simulink model "RBD"  (R2022a)
settings: Solver=VariableStepAuto  StartTime=0.0  StopTime=10.0  RelTol=1e-3
undefined symbols (not defined in the file or in its folder): dragConstants, g, J, J_inv, m, projectionMatrix
libraries: matrix_library x1, aerolibutil x1, sharedtransform x1
settings Model: Creator=Drew Lab Computer 1  LastModifiedBy=Drew Lab Computer 1

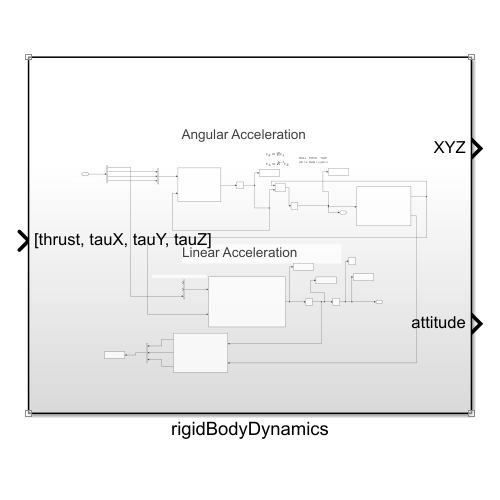
[thumbnail: Simulink's stored preview of the top-level diagram]
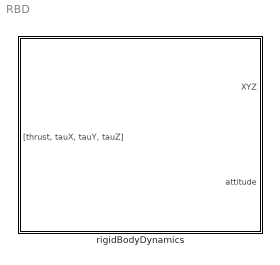
== system RBD ==
  rigidBodyDynamics : Subsystem

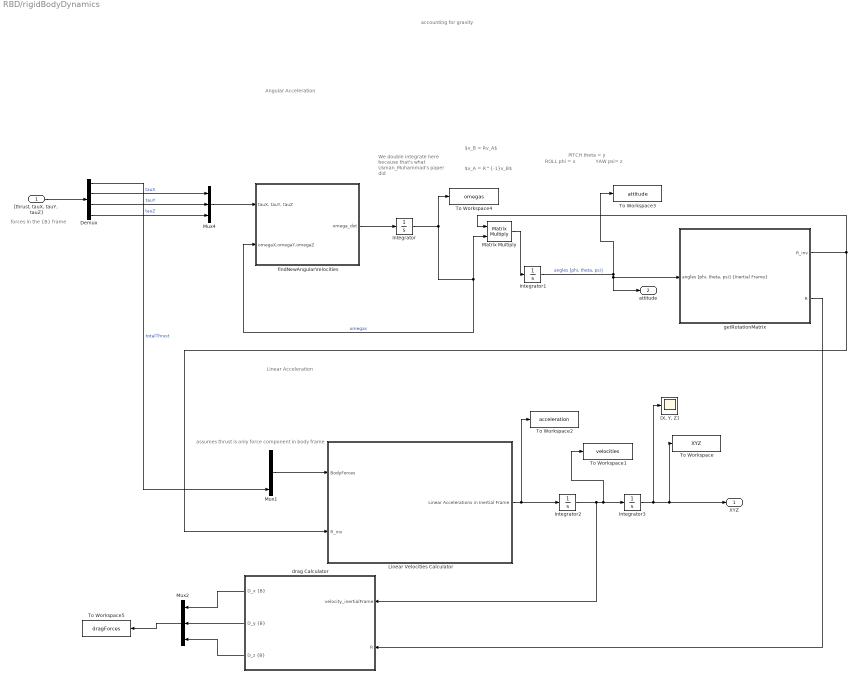
== system RBD/rigidBodyDynamics ==
  note: $v_A = R^{-1}v_B$
  note: assumes thrust is only force component in body frame
  note: We double integrate here because that's what Usman_Muhammad's paper did
  note: Angular Acceleration
  note: Linear Acceleration
  note: accounting for gravity
  note: forces in the {B} frame
  note: ROLL
      | phi = x
  note: PITCH
      | theta = y
  note: YAW
      | psi= z
  note: $v_B = Rv_A$
  "[thrust, tauX, tauY, tauZ]" : Inport
  Demux : Demux
  Integrator{,1..3} (4 alike) : Integrator
  Linear Velocities Calculator : Subsystem
  Matrix Multiply : Product  Multiplication=Matrix(*)
  Mux1 : Mux  Inputs=3
  Mux2 : Mux  Inputs=3
  Mux4 : Mux  Inputs=3
  To Workspace : ToWorkspace  VariableName=XYZ  SaveFormat=Timeseries  SampleTime=-1
  To Workspace1 : ToWorkspace  VariableName=velocities  SaveFormat=Timeseries  SampleTime=-1
  To Workspace2 : ToWorkspace  VariableName=acceleration  SaveFormat=Timeseries  SampleTime=-1
  To Workspace3 : ToWorkspace  VariableName=attitude  SaveFormat=Timeseries  SampleTime=-1
  To Workspace4 : ToWorkspace  VariableName=omegas  SaveFormat=Timeseries  SampleTime=-1
  To Workspace5 : ToWorkspace  VariableName=dragForces  SaveFormat=Timeseries  SampleTime=-1
  "[X, Y, Z]" : Scope
  drag Calculator : Subsystem
  findNewAngularVelocities : Subsystem
  getRotationMatrix : Subsystem
  XYZ : Outport
  attitude : Outport  Port=2
  wires:
  Demux/2 -> Mux4/1  "tauX"
  Demux/4 -> Mux4/3  "tauZ"
  Demux/3 -> Mux4/2  "tauY"
  "[thrust, tauX, tauY, tauZ]"/1 -> Demux/1
  Integrator1/1 -> attitude/1, getRotationMatrix/1("angles [phi, theta, psi] {Inertial Frame}"), To Workspace3/1  "angles [phi, theta, psi]"
  findNewAngularVelocities/1(omega_dot) -> Integrator/1
  Integrator/1 -> Matrix Multiply/2, findNewAngularVelocities/2(omegaX,omegaY,omegaZ), To Workspace4/1  "omegas"
  Mux4/1 -> findNewAngularVelocities/1("tauX, tauY, tauZ")
  Mux1/1 -> Linear Velocities Calculator/1(BodyForces)
  getRotationMatrix/1(R_inv) -> Linear Velocities Calculator/2(R_inv), Matrix Multiply/1
  Demux/1 -> Mux1/3  "totalThrust"
  Matrix Multiply/1 -> Integrator1/1
  Linear Velocities Calculator/1(Linear Accelerations in Inertial Frame) -> Integrator2/1, To Workspace2/1
  Integrator2/1 -> drag Calculator/1(velocity_inertialFrame), To Workspace1/1, Integrator3/1
  Integrator3/1 -> "[X, Y, Z]"/1, To Workspace/1, XYZ/1
  getRotationMatrix/2(R) -> drag Calculator/2(R)
  drag Calculator/2("D_y {B}") -> Mux2/2
  drag Calculator/1("D_x {B}") -> Mux2/1
  drag Calculator/3("D_z {B}") -> Mux2/3
  Mux2/1 -> To Workspace5/1

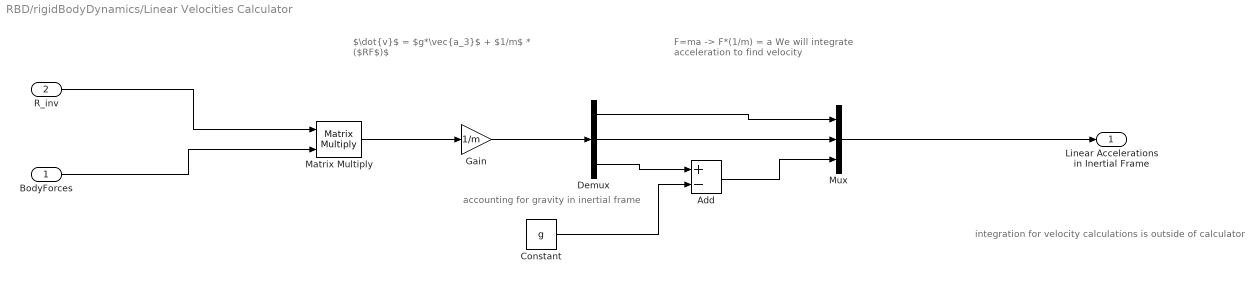
== system RBD/rigidBodyDynamics/Linear Velocities Calculator ==
  note: integration for velocity calculations is outside of calculator
  note: F=ma -> F*(1/m) = a
      | We will integrate acceleration to find velocity
  note: accounting for gravity in inertial frame
  note: $\dot{v}$ = $g*\vec{a_3}$ + $1/m$ * ($RF$)$
  BodyForces : Inport
  R_inv : Inport  Port=2
  Add : Sum  Inputs=+-
  Constant : Constant  Value=g
  Demux : Demux  Outputs=3
  Gain : Gain  Gain=1/m
  Matrix Multiply : Product  Multiplication=Matrix(*)
  Mux : Mux  Inputs=3
  Linear Accelerations in Inertial Frame : Outport
  wires:
  BodyForces/1 -> Matrix Multiply/2
  R_inv/1 -> Matrix Multiply/1
  Matrix Multiply/1 -> Gain/1
  Gain/1 -> Demux/1
  Demux/3 -> Add/1
  Add/1 -> Mux/3
  Demux/2 -> Mux/2
  Demux/1 -> Mux/1
  Mux/1 -> Linear Accelerations in Inertial Frame/1
  Constant/1 -> Add/2

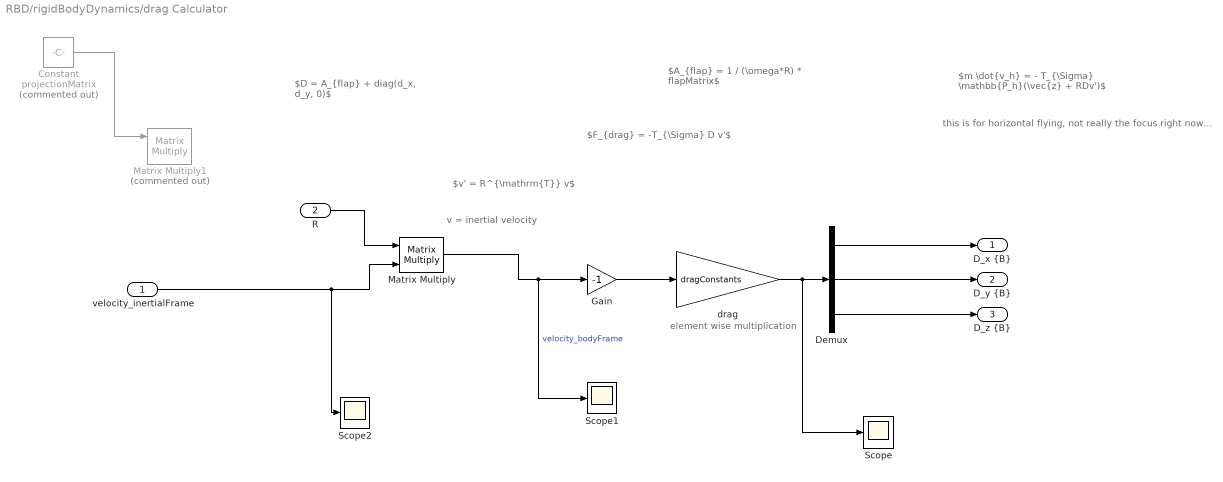
== system RBD/rigidBodyDynamics/drag Calculator ==
  note: element wise multiplication
  note: $A_{flap} = 1 / (\omega*R) * flapMatrix$
  note: $D = A_{flap} + diag(d_x, d_y, 0)$
  note: this is for horizontal flying, not really the focus right now...
  note: $F_{drag} = -T_{\Sigma} D v'$
  note: v = inertial velocity
  note: $v' = R^{\mathrm{T}} v$
  note: $m \dot{v_h} = - T_{\Sigma} \mathbb{P_h}(\vec{z} + RDv')$
  velocity_inertialFrame : Inport
  R : Inport  Port=2
  Constant : Constant  Commented=on  Value=projectionMatrix
  Demux : Demux  Outputs=3
  Gain : Gain  Gain=-1
  Matrix Multiply : Product  Multiplication=Matrix(*)
  Matrix Multiply1 : Product  Commented=on  Multiplication=Matrix(*)
  Scope : Scope
  Scope1 : Scope
  Scope2 : Scope
  drag : Gain  Gain=dragConstants
  "D_x {B}" : Outport
  "D_y {B}" : Outport  Port=2
  "D_z {B}" : Outport  Port=3
  wires:
  Matrix Multiply/1 -> Scope1/1, Gain/1  "velocity_bodyFrame"
  R/1 -> Matrix Multiply/1
  Demux/1 -> "D_x {B}"/1
  Demux/3 -> "D_z {B}"/1
  Gain/1 -> drag/1
  Constant/1 -> Matrix Multiply1/1
  drag/1 -> Scope/1, Demux/1
  Demux/2 -> "D_y {B}"/1
  velocity_inertialFrame/1 -> Scope2/1, Matrix Multiply/2

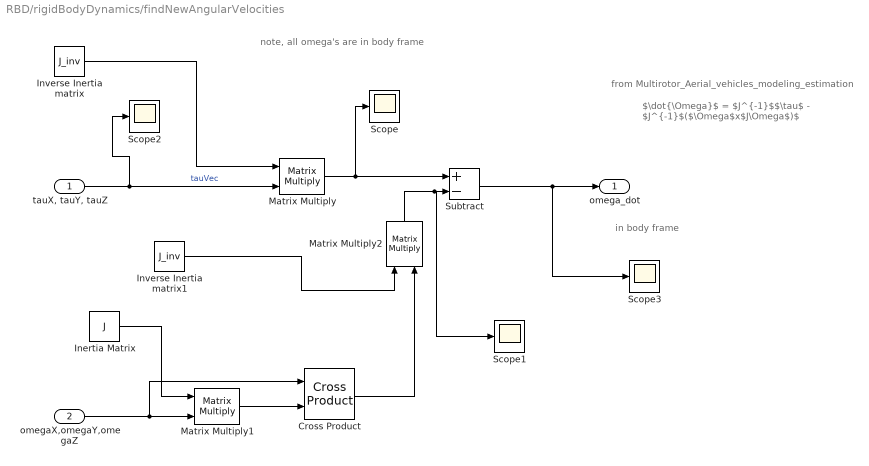
== system RBD/rigidBodyDynamics/findNewAngularVelocities ==
  note: from Multirotor_Aerial_vehicles_modeling_estimation
  note: note, all omega's are in body frame
  note: $\dot{\Omega}$ = $J^{-1}$$\tau$ - $J^{-1}$($\Omega$x$J\Omega$)$
  note: in body frame
  "tauX, tauY, tauZ" : Inport
  omegaX,omegaY,omegaZ : Inport  Port=2
  Cross Product : matrix_library/Cross Product
      settings: SourceProductBaseCode=SL
  Inertia Matrix : Constant  Value=J
  Inverse Inertia matrix : Constant  Value=J_inv
  Inverse Inertia matrix1 : Constant  Value=J_inv
  Matrix Multiply : Product  Multiplication=Matrix(*)
  Matrix Multiply1 : Product  Multiplication=Matrix(*)
  Matrix Multiply2 : Product  Multiplication=Matrix(*)
  Scope{,1..3} (4 alike) : Scope
  Subtract : Sum  Inputs=+-
  omega_dot : Outport
  wires:
  "tauX, tauY, tauZ"/1 -> Scope2/1, Matrix Multiply/2  "tauVec"
  Matrix Multiply/1 -> Scope/1, Subtract/1
  Inverse Inertia matrix/1 -> Matrix Multiply/1
  Inertia Matrix/1 -> Matrix Multiply1/1
  omegaX,omegaY,omegaZ/1 -> Cross Product/1, Matrix Multiply1/2
  Matrix Multiply1/1 -> Cross Product/2
  Inverse Inertia matrix1/1 -> Matrix Multiply2/1
  Cross Product/1 -> Matrix Multiply2/2
  Matrix Multiply2/1 -> Scope1/1, Subtract/2
  Subtract/1 -> Scope3/1, omega_dot/1

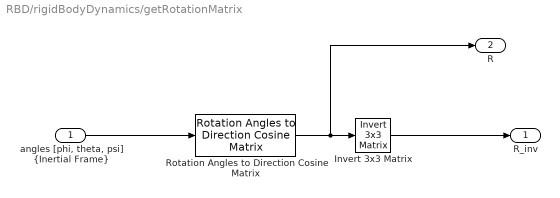
== system RBD/rigidBodyDynamics/getRotationMatrix ==
  "angles [phi, theta, psi] {Inertial Frame}" : Inport
  Invert 3x3 Matrix : aerolibutil/Invert  3x3 Matrix
  Rotation Angles to Direction Cosine Matrix : sharedtransform/Rotation Angles to Direction Cosine Matrix  rotationOrder=XYZ  aMode=aMode
      settings: SourceProductBaseCode=AE,PW,DR,MT,VE
  R_inv : Outport
  R : Outport  Port=2
  wires:
  "angles [phi, theta, psi] {Inertial Frame}"/1 -> Rotation Angles to Direction Cosine Matrix/1
  Rotation Angles to Direction Cosine Matrix/1 -> R/1, Invert 3x3 Matrix/1
  Invert 3x3 Matrix/1 -> R_inv/1
